simulink model "Moteur_Asynchrone_Base2019bG"  (R2020a)
settings: Solver=ode23tb  StartTime=0.0  StopTime=1.0  RelTol=1e-3  EnableMultiTasking=on
StopFcn:
  | sc = str2double(get_param('Moteur_Asynchrone_Base2019bG/Scenario_TP1','Value'));
  | try
  |   if ~evalin('base','exist(''simout'',''var'')'), return; end
  |   d = evalin('base','simout');
  |   switch round(sc)
  |     case 1, assignin('base','data_healthy', d);
  |     case 2, assignin('base','data_fault', d);
  |     case 3, assignin('base','data_fault_bearing', d);
  |   end
  | catch, end
libraries: powerlib x4
settings Model: Creator=NDJE  LastModifiedBy=RONALD TATCHEMO
settings SolverCC: ConcurrentTasks=on  AutoInsertRateTranBlk=on  InsertRTBMode=Never (minimum delay)
settings DataIOCC: SaveFormat=StructureWithTime  OutputSaveName=out
settings OptimizationCC: BlockReduction=off  OptimizeBlockIOStorage=off
settings HardwareCC: ProdBitPerPointer=32  ProdBitPerSizeT=32  ProdBitPerPtrDiffT=32  ProdLargestAtomicFloat=None  ProdWordSize=32  ProdLongLongMode=on  ProdHWDeviceType=Generic->32-bit x86 compatible
settings RTWCC: Description=Generic Real-Time Target  RTWCompilerOptimization=on
settings GRTTargetCC: TargetLangStandard=C89/C90 (ANSI)

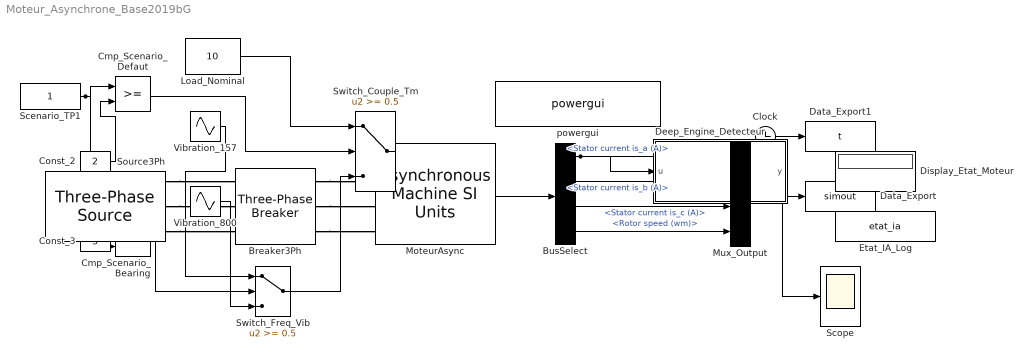
== system Moteur_Asynchrone_Base2019bG ==
  Breaker3Ph : powerlib/Elements/Three-Phase Breaker  InitialState=closed  SwitchA=on  SwitchB=on  SwitchC=on  SwitchTimes="[1/50  5/50]"  External=off  BreakerResistance=0.01  SnubberResistance=1  SnubberCapacitance=inf  Measurements=None
  BusSelect : BusSelector  OutputSignals=Stator measurements.Stator current is_a (A),Stator measurements.Stator current is_b (A),Stator measurements.Stator current is_c (A),Mechanical.Rotor speed (wm)
  Clock : Clock
  Cmp_Scenario_Bearing : RelationalOperator  OutDataTypeStr=boolean  RndMeth=Simplest
  Cmp_Scenario_Defaut : RelationalOperator  OutDataTypeStr=boolean  RndMeth=Simplest
  Const_2 : Constant  Value=2
  Const_3 : Constant  Value=3
  Data_Export : ToWorkspace  VariableName=simout  SaveFormat=Structure With Time  SampleTime=-1
  Data_Export1 : ToWorkspace  VariableName=t  SaveFormat=Structure With Time  SampleTime=-1
  Deep_Engine_Detecteur : MATLAB Function  TreatAsAtomicUnit=on
  Display_Etat_Moteur : Display
  Etat_IA_Log : ToWorkspace  VariableName=etat_ia  SampleTime=-1
  Load_Nominal : Constant  Value=10
  MoteurAsync : powerlib/Machines/Asynchronous Machine SI Units  RotorType=Squirrel-cage  PresetModel=No  MechanicalLoad=Torque Tm  ShowDetailedParameters=on  ReferenceFrame=Rotor  Units=SI  MeasurementBus=off  NominalParameters=[1.845e+04 400 50]  Stator=[0.435 0.002]  Rotor=[0.816 0.002]  Cage1=[0.4155 0.002066]  Cage2=[0.4168 0.0003495]  Lm=0.069  Mechanical=[0.89 0.005879 2]  PolePairs=2  InitialConditions=[0 0 0 0 0 0 0 0]  SimulateSaturation=off  Saturation=[14.03593122, 27.81365428, 53.79336849, 72.68890987, 97.98006896, 148.6815601, 215.7428561, 302.9841135, 428.7778367 ; 230, 322, 414, 460, 506, 552, 598, 644, 690]  LoadFlowParameters=1492000  TsPowergui=0  TsBlock=-1  IterativeModel=Trapezoidal non iterative  IterativeDiscreteModel=Trapezoidal non iterative  Pmec=1.492e+006
  Mux_Output : Mux
  Scenario_TP1 : Constant
  Scope : Scope
  Source3Ph : powerlib/Electrical Sources/Three-Phase Source  InternalConnection=Yg  VoltagePhases=off  Voltage=380  PhaseAngle=0  Voltage_phases=[25e3 25e3 25e3]/sqrt(3)  PhaseAngles_phases=[0 -120 +120]  Frequency=50  NonIdealSource=on  SpecifyImpedance=off  Resistance=0.8929  Inductance=0  ShortCircuitLevel=100e6  BaseVoltage=380  XRratio=7  BusType=swing  Pref=10e3  Qref=0  Prefabc=[10e3, 10e3, 10e3]  Qrefabc=[0, 0, 0]  Qmin=-inf  Qmax=inf
  Switch_Couple_Tm : Switch  Threshold=0.5
  Switch_Freq_Vib : Switch  Threshold=0.5
  Vibration_157 : Sin  Amplitude=5  Frequency=157  SampleTime=0
  Vibration_800 : Sin  Amplitude=5  Frequency=800  SampleTime=0
  powergui : powerlib/powergui  Priority=1  SimulationMode=Discrete  SampleTime=50e-6  frequency=60  Iterations=50  frequencyindice=50  Pbase=100e6  ErrMax=1e-4  UnitsV=kV  UnitsW=MW  buscounter=0  FunctionMessages=off  echomessages=off  EnableUseOfTLC=off  CurrentSourceSwitches=on  DisableSnubberDevices=off  DisableRonSwitches=off  DisableVfSwitches=off  DisplayEquations=off  AutomaticDiscreteSolvers=off  SolverType=Tustin/Backward Euler (TBE)  Interpol=off  ExternalGateDelay=off  methode=off  Ts=100  x0status=blocks  SPID=on  SwTol=0  HookPort=off  NonlinearTolerance=1e-4  nMaxIteration=100  ContinueOnMaxIteration=off  RestoreLinks=warning  ResistiveCurrentMeasurement=off  Frange=[0:2:500]  Ylog=off  Xlog=on  ShowGrid=off  save=off  variable=ZData  structure=0  ZoomFFT=off  StartTime=0.0  cycles=1  DisplayStyle=1  fundamental=60  FreqAxis=off  MaxFrequency=1000  frequencyindicesteady=1  RmsSteady=1  display=off
  wires:
  MoteurAsync/1 -> BusSelect/1
  BusSelect/1 -> Mux_Output/1, Deep_Engine_Detecteur/1(u)  "<Stator current is_a (A)>"
  BusSelect/2 -> Mux_Output/2  "<Stator current is_b (A)>"
  BusSelect/3 -> Mux_Output/3  "<Stator current is_c (A)>"
  BusSelect/4 -> Mux_Output/4  "<Rotor speed (wm)>"
  Mux_Output/1 -> Scope/1, Data_Export/1
  Clock/1 -> Data_Export1/1
  Scenario_TP1/1 -> Cmp_Scenario_Defaut/1, Cmp_Scenario_Bearing/1
  Const_2/1 -> Cmp_Scenario_Defaut/2
  Const_3/1 -> Cmp_Scenario_Bearing/2
  Vibration_157/1 -> Switch_Freq_Vib/1
  Cmp_Scenario_Bearing/1 -> Switch_Freq_Vib/2
  Vibration_800/1 -> Switch_Freq_Vib/3
  Load_Nominal/1 -> Switch_Couple_Tm/1
  Cmp_Scenario_Defaut/1 -> Switch_Couple_Tm/2
  Switch_Freq_Vib/1 -> Switch_Couple_Tm/3
  Switch_Couple_Tm/1 -> MoteurAsync/1
  ? -> Display_Etat_Moteur/1, Etat_IA_Log/1
  connections:
  Source3Ph/RConn1 -- Breaker3Ph/LConn1
  Source3Ph/RConn2 -- Breaker3Ph/LConn2
  Source3Ph/RConn3 -- Breaker3Ph/LConn3
  Breaker3Ph/RConn1 -- MoteurAsync/LConn1
  Breaker3Ph/RConn2 -- MoteurAsync/LConn2
  Breaker3Ph/RConn3 -- MoteurAsync/LConn3

== matlab function Moteur_Asynchrone_Base2019bG/Deep_Engine_Detecteur ==
  data: u input; y output
function y = fcn(u)

y = u;
